simulink model "kararmekanizmasideneme"  (R2020b)
settings: Solver=VariableStepAuto  StartTime=0.0  StopTime=180  RelTol=1e-3
libraries: aerolibanimutils x1
settings Model: Creator=tkara  LastModifiedBy=tkara

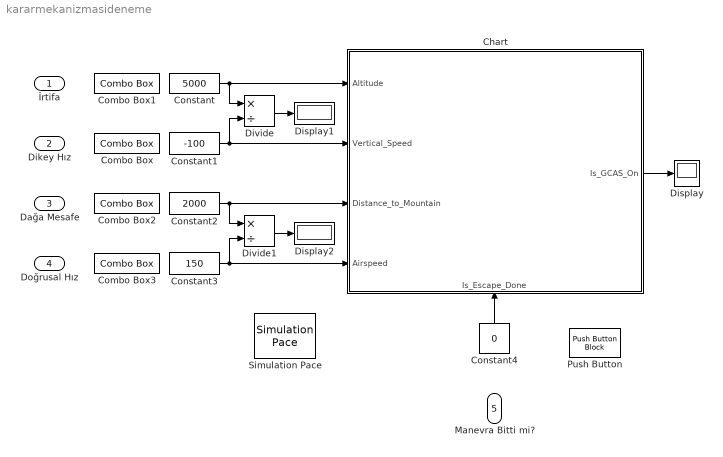
== system kararmekanizmasideneme ==
  İrtifa : Inport
  Dikey Hız : Inport  Port=2
  Dağa Mesafe : Inport  Port=3
  Doğrusal Hız : Inport  Port=4
  Manevra Bitti mi? : Inport  Port=5
  Chart : Stateflow chart  TreatAsAtomicUnit=on
      settings: PortSchema="{\"entries\":[{\"content\":{\"sides\":[{\"content\":{\"connectorIds\":[\"In1\",\"In2\",\"In3\",\"In4\"]},\"type\":\"ConnectorPlacement.EquallySpacedRectSide\",\"uuid\":\"ff2c2f4c-49f1-4bbe-9488-7760f3f308d8\"},{\"content\":{\"connectorIds\":[\"Out1\"],\"side\":\"RIGHT\"},\"type\":\"ConnectorPlacement.EquallySpacedRectSide\",\"uuid\":\"affa6758-c02a-42eb-b092-4a2ea7a7333a\"},{\"content\":{\"connectorIds\":[],\"side\":\"TOP\"},\"type\":\"ConnectorPlacement.EquallySpacedRectSide\",\"uuid\":\"f2917a35-03fa-4c14-9824-44541cf3d2c0\"},{\"content\":{\"connectorIds\":[\"In5\"],\"side\":\"BOTTOM\"},\"type\":\"ConnectorPlacement.EquallySpacedRectSide\",\"uuid\":\"b0f4133c-bb13-4dbd-8543-7cfc0b137815\"},{\"content\":{\"connectorIds\":[],\"side\":\"HIDDEN\"},\"type\":\"ConnectorPlacement.EquallySpacedRectSide\",\"uuid\":\"caae7eb5-e2db-45d7-a64a-9fce692b7805\"}]},\"type\":\"ConnectorPlacement.EquallySpacedConnector\",\"uuid\":\"a226d3be-ad19-4fbe-a7f9-0a8466de4f24\"}],\"packageUris\":[\"http://schema.mathworks.com/mf0/Connector/R2020b\"],\"version\":\"1.0\"}"
  Combo Box : ComboBox  LabelPosition=Hide  SelectedLabel=Diving
      settings: Values={{'Level Flight', 'Descending', 'Diving'}, [0 -50 -100]}
  Combo Box1 : ComboBox  LabelPosition=Hide  SelectedLabel=High Alt.
      settings: Values={{'Ground', 'Low Alt.', 'High Alt.'}, [0 400 5000]}
  Combo Box2 : ComboBox  LabelPosition=Hide  SelectedLabel=Far
      settings: Values={{'Boom', 'Close', 'Far'}, [0 200 2000]}
  Combo Box3 : ComboBox  LabelPosition=Hide  SelectedLabel=Low Speed
      settings: Values={{'Zero', 'Low Speed', 'High Speed'}, [50 150 360]}
  Constant : Constant  Value=5000
  Constant1 : Constant  Value=-100
  Constant2 : Constant  Value=2000
  Constant3 : Constant  Value=150
  Constant4 : Constant  Value=0
  Display : Display
  Display1 : Display
  Display2 : Display
  Divide : Product  Inputs=*/
  Divide1 : Product  Inputs=*/
  Push Button : PushButtonBlock
  Simulation Pace : aerolibanimutils/Simulation Pace  SimulationPace=1  SleepMode=Auto  OutputPaceError=off  SampleTime=1/30
  wires:
  Chart/1(Is_GCAS_On) -> Display/1
  Constant/1 -> Divide/1, Chart/1(Altitude)
  Constant1/1 -> Divide/2, Chart/2(Vertical_Speed)
  Constant4/1 -> Chart/5(Is_Escape_Done)
  Divide/1 -> Display1/1
  Divide1/1 -> Display2/1
  Constant3/1 -> Divide1/2, Chart/4(Airspeed)
  Constant2/1 -> Divide1/1, Chart/3(Distance_to_Mountain)

== stateflow chart kararmekanizmasideneme/Chart ==
  state Safe
    Is_GCAS_On = 0
  state Danger
    Is_GCAS_On = 1
  (default) -> Safe
  Danger -> Safe : [Is_Escape_Done==1]
  Safe -> Danger [order 1] : [(Distance_to_Mountain/Airspeed)<5]
  Safe -> Danger [order 2] : [(Altitude/-Vertical_Speed)<5]
  data: Altitude input; Vertical_Speed input; Distance_to_Mountain input; Airspeed input; Is_Escape_Done input; Is_GCAS_On output
